simulink model "PatientSIMULATOR_MIMOnoNMB"  (R2022a)
settings: Solver=ode4  StartTime=0.0  StopTime=info.Tsim  FixedStep=0.1  RelTol=1e-15
values from neighbouring files (symbols this model uses):
  condDiscMat = BuildCondendsedMPCmatrices(discreteMat,r,q,F,f,PH)    [MAIN_MIMO.m]    (also in backupMain.m; test.m)
  discreteModel = c2d(continuousModel, info.Ts)    [MAIN_MIMO.m]    (also in backupMain.m; nonLinearPatient_main.m; test.m)
  kalmDiscMat = BuildCondendsedMPCmatrices(discreteMat,r_Kalman,q_Kalman,F,f,PH)    [MAIN_MIMO.m]    (also in test.m)
  PH = 200    [MAIN_MIMO.m]    (also in backupMain.m; nonLinearPatient_main.m; test.m)
  R_KF = 0.001*eye(2)    [MAIN_MIMO.m]    (also in backupMain.m; nonLinearPatient_main.m; test.m)
  wantNoisyBIS = 1    [MAIN_MIMO.m]    (also in backupMain.m; nonLinearPatient_main.m; test.m)
  x_eq = operatingPoint.getstatestruct.signals.values    [MAIN_MIMO.m]    (also in backupMain.m; nonLinearPatient_main.m; test.m)
undefined symbols (not defined in the file or in its folder): continuousModel, Discrete, info, myMPC_dist, op, patient, propofol, RASS, remifentanil, Time
libraries: ctrlSharedLib x3, cstblocks x2
settings Model: Creator=cionescu  LastModifiedBy=user
settings SolverCC: AlgebraicLoopSolver=TrustRegion
settings DataIOCC: SaveState=on  ReturnWorkspaceOutputs=off
settings DebuggingCC: UnconnectedInputMsg=warning  UnconnectedOutputMsg=warning  UnconnectedLineMsg=warning  SFMachineParentedDataDiag=warning  ArithmeticOperatorsInVariantConditions=warning
settings SFSimCC: SimUseLocalCustomCode=off  CustomCodeUndefinedFunction=UseInterfaceOnly
settings RTWCC: RTWUseLocalCustomCode=off  DLArmComputeVersion=19.05
settings CodeAppCC: StateflowObjectComments=on

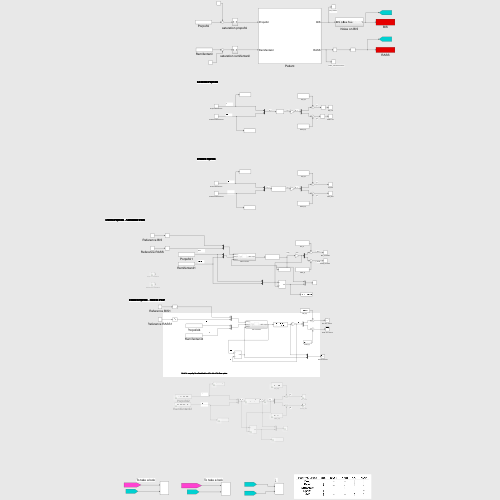
[thumbnail: Simulink's stored preview of the top-level diagram]
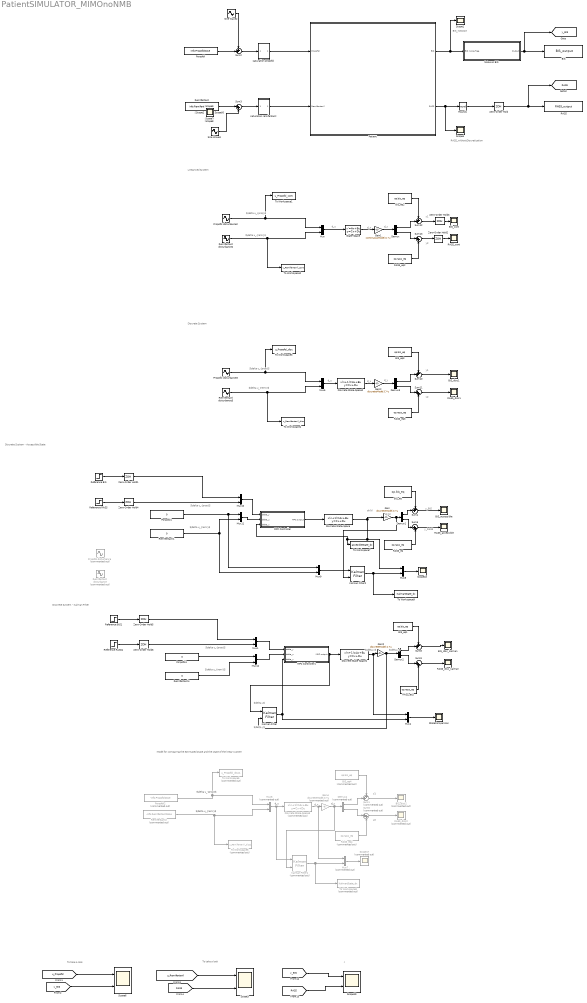
== system PatientSIMULATOR_MIMOnoNMB ==
  note: Model for comparing the estimated state and the state of the linear system
  note: RASS_withoutDiscretization
  note: BIS_noNoise
  note: y2
  note: y1
  note: d_u
  note: d_y
  note: d_x
  note: Linearized System
  note: ↓
  note: To take a look
  note: To take a look
  note: y2
  note: d_y
  note: y1
  note: d_u
  note: d_x
  note: Discrete System
  note: $\delta u_{remi}$
  note: $\delta u_{prop}$
  note: $\delta u_{remi}$
  note: $\delta u_{prop}$
  note: $\delta u_{remi}$
  note: dx(k)
  note: y_RASS
  note: Discrete System - Accessible State
  note: dy(k)
  note: y_BIS
  note: $\delta u_{prop}$
  note: $\delta y$
  note: $\delta x$
  note: $\delta y$
  note: $\delta u$
  note: Discrete System - Kalman Filter
  note: d_u
  note: $\delta u_{remi}$
  note: $\delta u_{prop}$
  note: y1
  note: d_y
  note: y2
  note: d_x
  note: $\delta u_{prop}$
  note: $\delta u_{remi}$
  BIS : ToWorkspace  VariableName=BIS_output  SampleTime=1
      settings: Save2DSignal=2-D array (concatenate along first dimension)
  BIS_accessible : Scope
  BIS_cont : Scope
  BIS_disc1 : Scope
  BIS_disc2 : Scope  Commented=on
  BIS_disc_kalman : Scope
  BIS_eq : Constant  Value=op.bis_eq
  BIS_eq1 : Constant  Value=op.bis_eq
  BIS_eq2 : Constant  Value=op.bis_eq
  BIS_eq3 : Constant  Value=op.bis_eq  SampleTime=info.Ts
  BIS_eq4 : Constant  Commented=on  Value=op.bis_eq  SampleTime=info.Ts
  Demux{,1..3} (4 alike) : Demux  Outputs=2
  Demux4 : Demux  Commented=on  Outputs=2
  Discrete State-Space : DiscreteStateSpace  A=discreteModel.A  B=discreteModel.B  C=eye(size(discreteModel.A))  D=zeros(size(discreteModel.A,1),size(discreteModel.B,2))  InitialCondition=[0,0,0,-0.5584,-2,0,0,0,0,0]'  SampleTime=info.Ts
  Discrete State-Space1 : DiscreteStateSpace  A=discreteModel.A  B=discreteModel.B  C=eye(size(discreteModel.A))  D=zeros(size(discreteModel.A,1),size(discreteModel.B,2))  InitialCondition=[0,0,0,-0.5584,-2,0,0,0,0,0]  SampleTime=info.Ts
  Discrete State-Space2 : DiscreteStateSpace  A=discreteModel.A  B=discreteModel.B  C=eye(size(discreteModel.A))  D=zeros(size(discreteModel.A,1),size(discreteModel.B,2))  InitialCondition=[0,0,0,-0.5584,-2,0,0,0,0,0]'  SampleTime=info.Ts
  Discrete State-Space3 : DiscreteStateSpace  Commented=on  A=discreteModel.A  B=discreteModel.B  C=eye(size(discreteModel.A))  D=zeros(size(discreteModel.A,1),size(discreteModel.B,2))  SampleTime=info.Ts
  Gain : Gain  Gain=discreteModel.C  Multiplication=Matrix(K*u)
  Gain1 : Gain  Gain=continuousModel.C  Multiplication=Matrix(K*u)
  Gain2 : Gain  Gain=discreteModel.C  Multiplication=Matrix(K*u)
  Gain3 : Gain  Gain=discreteModel.C  Multiplication=Matrix(K*u)
  Gain4 : Gain  Commented=on  Gain=discreteModel.C  Multiplication=Matrix(K*u)
  Kalman Filter : ctrlSharedLib/Kalman Filter  TimeDomain=Discrete-Time  UseCurrentEstimator=on  ModelSource=LTI State-Space Variable  ModelSourceVariable=discreteModel  A=0.95  B=1  C=1  D=0  NumberOfStates=1  NumberOfInputs=1  NumberOfOutputs=1  InitialEstimateSource=Dialog  X0=x_eq  P0=10  UseK=off  UseGH=off  NumberOfProcessNoiseInputs=1  G=1  TimeInvariantG=on  H=0  TimeInvariantH=on  Q=Q_KF  TimeInvariantQ=on  R=R_KF  TimeInvariantR=on  N=0  TimeInvariantN=on  AddInputPort=on  AddEnablePort=off  OutputEstimatedY=off  OutputP=off  Ts=-1
  Kalman Filter1 : ctrlSharedLib/Kalman Filter  Commented=on  TimeDomain=Discrete-Time  UseCurrentEstimator=on  ModelSource=LTI State-Space Variable  ModelSourceVariable=discreteModel  A=0.95  B=1  C=1  D=0  NumberOfStates=1  NumberOfInputs=1  NumberOfOutputs=1  InitialEstimateSource=Dialog  X0=[0,0,0,-0.5584,-2,0,0,0,0,0]  P0=10  UseK=off  UseGH=off  NumberOfProcessNoiseInputs=1  G=1  TimeInvariantG=on  H=0  TimeInvariantH=on  Q=Q_KF  TimeInvariantQ=on  R=R_KF  TimeInvariantR=on  N=0  TimeInvariantN=on  AddInputPort=on  AddEnablePort=off  OutputEstimatedY=off  OutputP=off  Ts=-1
  Kalman Filter2 : ctrlSharedLib/Kalman Filter  TimeDomain=Discrete-Time  UseCurrentEstimator=on  ModelSource=LTI State-Space Variable  ModelSourceVariable=discreteModel  A=0.95  B=1  C=1  D=0  NumberOfStates=1  NumberOfInputs=1  NumberOfOutputs=1  InitialEstimateSource=Dialog  X0=[0,0,0,-0.5584,-2,0,0,0,0,0]'  P0=10  UseK=off  UseGH=off  NumberOfProcessNoiseInputs=1  G=1  TimeInvariantG=on  H=0  TimeInvariantH=on  Q=Q_KF  TimeInvariantQ=on  R=R_KF  TimeInvariantR=on  N=0  TimeInvariantN=on  AddInputPort=on  AddEnablePort=off  OutputEstimatedY=off  OutputP=off  Ts=-1
  MPC Controller : Subsystem
  MPC Controller1 : Subsystem
  Mux{,1,4..5,8..12} (9 alike) : Mux  Inputs=2
  Mux6 : Mux  Commented=on  Inputs=2
  Mux7 : Mux  Commented=on  Inputs=2
  Noise on BIS : Subsystem
  Patient : Subsystem
  Porpofol : Constant  Value=info.PropofolDose  SampleTime=info.Ts
  Porpofol1 : Constant  Value=0  SampleTime=info.Ts
  Porpofol2 : Constant  Commented=on  Value=-info.PropofolDose  SampleTime=info.Ts
  Porpofol4 : Constant  Value=0  SampleTime=info.Ts
  Propofol disturbance : Sin  Commented=on  Amplitude=0.3*op.propofol_eq  Frequency=1/500  SampleTime=info.Ts
  Propofol disturbance2 : Sin  Amplitude=0.3*op.propofol_eq  Frequency=1/500  SampleTime=0
  Propofol disturbance3 : Sin  Amplitude=0.3*op.propofol_eq  Frequency=1/500  SampleTime=info.Ts
  RASS : ToWorkspace  VariableName=RASS_output  SampleTime=1
      settings: Save2DSignal=2-D array (concatenate along first dimension)
  RASS_accessible : Scope
  RASS_cont : Scope
  RASS_disc1 : Scope
  RASS_disc2 : Scope  Commented=on
  RASS_disc_kalman : Scope
  RASS_eq : Constant  Value=op.rass_eq
  RASS_eq1 : Constant  Value=op.rass_eq
  RASS_eq2 : Constant  Value=op.rass_eq
  RASS_eq3 : Constant  Value=op.rass_eq  SampleTime=info.Ts
  RASS_eq4 : Constant  Commented=on  Value=op.rass_eq  SampleTime=info.Ts
  Reference BIS : Step  Time=info.T_induction  Before=50  After=0  SampleTime=info.Ts
  Reference BIS1 : Step  Time=info.T_induction  Before=50  After=0  SampleTime=info.Ts
  Reference RASS : Step  Time=info.T_induction  Before=4  After=0  SampleTime=info.Ts
  Reference RASS1 : Step  Time=info.T_induction  Before=4  After=0  SampleTime=info.Ts
  Remifentanil : Constant  Value=info.RemifentanilDose  SampleTime=info.Ts
  Remifentanil disturbance : Sin  Commented=on  Amplitude=0.3*op.remifentanil_eq  Frequency=1/700  SampleTime=info.Ts
  Remifentanil disturbance2 : Sin  Amplitude=0.3*op.remifentanil_eq  Frequency=1/700  SampleTime=0
  Remifentanil disturbance3 : Sin  Amplitude=0.3*op.remifentanil_eq  Frequency=1/700  SampleTime=info.Ts
  Remifentanil1 : Constant  Value=0  SampleTime=info.Ts
  Remifentanil2 : Constant  Commented=on  Value=-info.RemifentanilDose  SampleTime=info.Ts
  Remifentanil4 : Constant  Value=0  SampleTime=info.Ts
  Round1 : Rounding  Operator=round
  Scope{,1..2,4..5,7..16,18} (16 alike) : Scope
  Scope17 : Scope  Commented=on
  Scope19 : Scope  NumInputPorts=2
  Scope3 : Scope  NumInputPorts=2
  Scope6 : Scope  NumInputPorts=2
  Sine Wave2 : Sin  Amplitude=0.3*op.propofol_eq  Frequency=1/500  SampleTime=0
  Sine Wave3 : Sin  Amplitude=0.3*op.remifentanil_eq  Frequency=1/700  SampleTime=0
  State-Space : StateSpace  A=continuousModel.A  B=continuousModel.B  C=eye(size(continuousModel.A))  D=zeros(size(continuousModel.A,1),size(continuousModel.B,2))  InitialCondition=[0,0,0,-0.5584,-2,0,0,0,0,0]'
  StateComparison : Scope
  Sum1 : Sum  Commented=on  Inputs=++|
  Sum{2,4,8,10,12} (5 alike) : Sum  Inputs=++|
  Sum{3,5,9,11,13} (5 alike) : Sum  Inputs=|++
  Sum6 : Sum  Commented=on  Inputs=|++
  To Workspace1 : ToWorkspace  VariableName=u_Propofol_cont  SaveFormat=Structure With Time  SampleTime=-1
      settings: Save2DSignal=2-D array (concatenate along first dimension)
  To Workspace2 : ToWorkspace  VariableName=u_Remifentanil_cont  SaveFormat=Structure With Time  SampleTime=-1
      settings: Save2DSignal=2-D array (concatenate along first dimension)
  To Workspace3 : ToWorkspace  VariableName=u_Propofol_disc  SaveFormat=Structure With Time  SampleTime=info.Ts
      settings: Save2DSignal=2-D array (concatenate along first dimension)
  To Workspace4 : ToWorkspace  VariableName=u_Remifentanil_disc  SaveFormat=Structure With Time  SampleTime=info.Ts
      settings: Save2DSignal=2-D array (concatenate along first dimension)
  To Workspace5 : ToWorkspace  Commented=on  VariableName=u_Propofol_disc1  SaveFormat=Structure With Time  SampleTime=info.Ts
      settings: Save2DSignal=2-D array (concatenate along first dimension)
  To Workspace6 : ToWorkspace  Commented=on  VariableName=u_Remifentanil_disc1  SaveFormat=Structure With Time  SampleTime=info.Ts
      settings: Save2DSignal=2-D array (concatenate along first dimension)
  To Workspace7 : ToWorkspace  VariableName=accesibleState_dx  SaveFormat=Structure With Time  SampleTime=-1
  To Workspace8 : ToWorkspace  Commented=on  VariableName=KalmanState_dx  SaveFormat=Structure With Time  SampleTime=-1
  To Workspace9 : ToWorkspace  VariableName=KalmanState_dx  SaveFormat=Structure With Time  SampleTime=-1
  Zero-Order Hold{,1..6} (7 alike) : ZeroOrderHold  SampleTime=info.Ts
  "saturation propofol " : Subsystem
  saturation remifentanil : Subsystem
  tag scope: RASS=global, y_BIS=global
  wires:
  [u_Propofol] -> Scope6/1
  [y_BIS] -> Scope6/2
  [RASS] -> Scope3/2
  [u_Remifentanil] -> Scope3/1
  Round1/1 -> Zero-Order Hold/1
  [y_BIS] -> Scope19/1
  [RASS] -> Scope19/2
  Zero-Order Hold/1 -> [RASS], RASS/1
  Patient/1(BIS) -> Scope1/1, Noise on BIS/1(BIS noise free)
  Porpofol/1 -> Sum2/2
  "saturation propofol "/1(Out1) -> Patient/1(Propofol)
  Remifentanil/1 -> Sum3/1
  saturation remifentanil/1(Out1) -> Patient/2(Remifentanil)
  Patient/2(RASS) -> Scope4/1, Round1/1
  Noise on BIS/1(Output) -> [y_BIS], BIS/1
  Mux/1 -> State-Space/1
  Propofol disturbance2/1 -> Mux/1, To Workspace1/1
  Remifentanil disturbance2/1 -> To Workspace2/1, Mux/2
  State-Space/1 -> Gain1/1
  Demux/2 -> Sum13/1
  Sine Wave2/1 -> Sum2/1
  Sum2/1 -> "saturation propofol "/1(In1)
  Sine Wave3/1 -> Sum3/2
  Sum3/1 -> saturation remifentanil/1(In1)
  Demux/1 -> Sum12/2
  Gain1/1 -> Demux/1
  BIS_eq2/1 -> Sum12/1
  Sum12/1 -> Zero-Order Hold3/1
  RASS_eq2/1 -> Sum13/2
  Zero-Order Hold3/1 -> BIS_cont/1
  RASS_eq3/1 -> Sum11/2
  BIS_eq3/1 -> Sum10/1
  Propofol disturbance3/1 -> Mux5/1, To Workspace3/1
  Gain3/1 -> Demux3/1
  Demux3/1 -> Sum10/2
  Remifentanil disturbance3/1 -> To Workspace4/1, Mux5/2
  Mux5/1 -> Discrete State-Space2/1
  Demux3/2 -> Sum11/1
  Sum10/1 -> BIS_disc1/1
  Sum11/1 -> RASS_disc1/1
  Sum13/1 -> Zero-Order Hold2/1
  Zero-Order Hold2/1 -> RASS_cont/1
  BIS_eq/1 -> Sum4/1
  Demux1/2 -> Sum5/1
  RASS_eq/1 -> Sum5/2
  Demux1/1 -> Sum4/2
  BIS_eq1/1 -> Sum8/1
  MPC Controller1/1(MPC output) -> Kalman Filter/1, Discrete State-Space1/1
  Sum9/1 -> RASS_disc_kalman/1
  Discrete State-Space1/1 -> Gain2/1, Mux4/1
  RASS_eq1/1 -> Sum9/2
  Gain2/1 -> Demux2/1, Kalman Filter/2
  Sum8/1 -> BIS_disc_kalman/1
  Demux2/2 -> Sum9/1
  Mux4/1 -> StateComparison/1
  Demux2/1 -> Sum8/2
  Gain/1 -> Kalman Filter2/2, Demux1/1
  Discrete State-Space2/1 -> Gain3/1
  Sum5/1 -> RASS_accessible/1
  Sum4/1 -> BIS_accessible/1
  Demux4/2 -> Sum6/1
  Porpofol2/1 -> Mux6/1, To Workspace5/1
  Sum6/1 -> RASS_disc2/1
  Mux6/1 -> Kalman Filter1/1, Discrete State-Space3/1
  Demux4/1 -> Sum1/2
  Discrete State-Space3/1 -> Mux7/1, Gain4/1
  Remifentanil2/1 -> Mux6/2, To Workspace6/1
  Gain4/1 -> Kalman Filter1/2, Demux4/1
  Sum1/1 -> BIS_disc2/1
  RASS_eq4/1 -> Sum6/2
  BIS_eq4/1 -> Sum1/1
  Mux7/1 -> Scope17/1
  Kalman Filter1/1 -> To Workspace8/1, Mux7/2
  Discrete State-Space/1 -> Gain/1, MPC Controller/3(delta_x), To Workspace7/1, Mux8/1
  Mux8/1 -> Scope18/1
  Kalman Filter2/1 -> To Workspace9/1, Mux8/2
  Mux9/1 -> Kalman Filter2/1
  Porpofol1/1 -> Mux9/1, Mux11/1
  Remifentanil1/1 -> Mux9/2, Mux11/2
  Reference BIS/1 -> Zero-Order Hold1/1
  Reference RASS/1 -> Zero-Order Hold4/1
  Zero-Order Hold1/1 -> Mux10/1
  Zero-Order Hold4/1 -> Mux10/2
  Mux10/1 -> MPC Controller/1(delta_y)
  Mux11/1 -> MPC Controller/2(delta_u)
  MPC Controller/1(MPC output) -> Discrete State-Space/1
  Mux12/1 -> MPC Controller1/2(delta_u)
  Mux1/1 -> MPC Controller1/1(delta_y)
  Zero-Order Hold5/1 -> Mux1/1
  Reference BIS1/1 -> Zero-Order Hold5/1
  Remifentanil4/1 -> Mux12/2
  Zero-Order Hold6/1 -> Mux1/2
  Porpofol4/1 -> Mux12/1
  Kalman Filter/1 -> Mux4/2, MPC Controller1/3(delta_x)
  Reference RASS1/1 -> Zero-Order Hold6/1

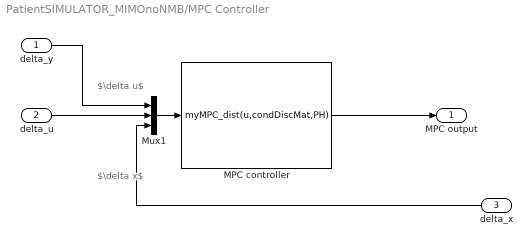
== system PatientSIMULATOR_MIMOnoNMB/MPC Controller ==
  note: $\delta x$
  note: $\delta u$
  delta_y : Inport
  delta_u : Inport  Port=2
  delta_x : Inport  Port=3
  MPC controller : MATLABFcn  MATLABFcn=myMPC_dist(u,condDiscMat,PH)  OutputDimensions=2
  Mux1 : Mux  Inputs=3
  MPC output : Outport
  wires:
  delta_x/1 -> Mux1/3
  Mux1/1 -> MPC controller/1
  MPC controller/1 -> MPC output/1
  delta_u/1 -> Mux1/2
  delta_y/1 -> Mux1/1

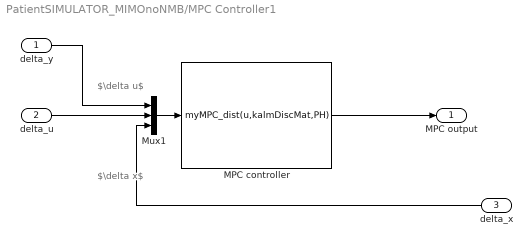
== system PatientSIMULATOR_MIMOnoNMB/MPC Controller1 ==
  note: $\delta x$
  note: $\delta u$
  delta_y : Inport
  delta_u : Inport  Port=2
  delta_x : Inport  Port=3
  MPC controller : MATLABFcn  MATLABFcn=myMPC_dist(u,kalmDiscMat,PH)  OutputDimensions=2
  Mux1 : Mux  Inputs=3
  MPC output : Outport
  wires:
  delta_x/1 -> Mux1/3
  Mux1/1 -> MPC controller/1
  MPC controller/1 -> MPC output/1
  delta_u/1 -> Mux1/2
  delta_y/1 -> Mux1/1

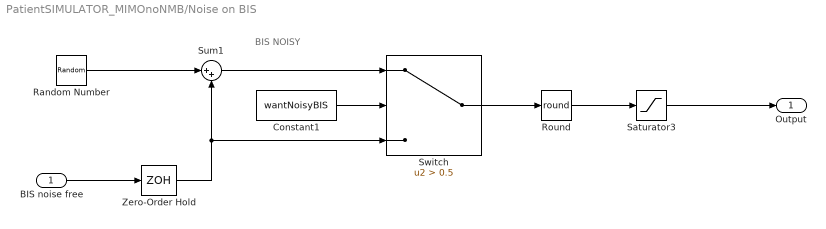
== system PatientSIMULATOR_MIMOnoNMB/Noise on BIS ==
  note: BIS NOISY
  BIS noise free : Inport
  Constant1 : Constant  Value=wantNoisyBIS
  Random Number : RandomNumber  Variance=6.27  SampleTime=info.Ts
  Round : Rounding  Operator=round
  Saturator3 : Saturate  UpperLimit=100  LowerLimit=0
  Sum1 : Sum  Inputs=|++
  Switch : Switch  Criteria=u2 > Threshold  Threshold=0.5  SaturateOnIntegerOverflow=off  InputSameDT=off
  Zero-Order Hold : ZeroOrderHold  SampleTime=info.Ts
  Output : Outport
  wires:
  Round/1 -> Saturator3/1
  Random Number/1 -> Sum1/1
  Constant1/1 -> Switch/2
  Saturator3/1 -> Output/1
  Switch/1 -> Round/1
  BIS noise free/1 -> Zero-Order Hold/1
  Sum1/1 -> Switch/1
  Zero-Order Hold/1 -> Sum1/2, Switch/3

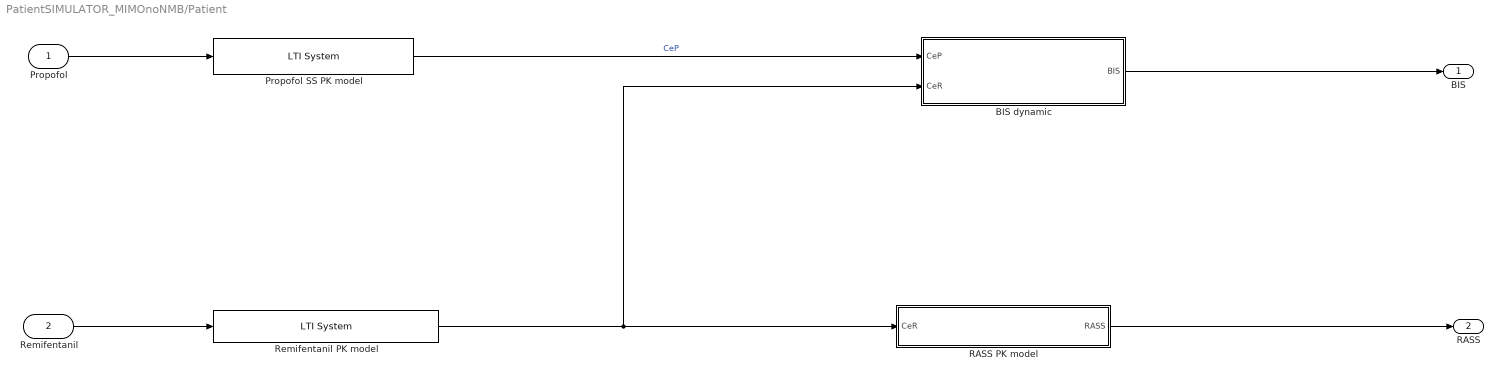
== system PatientSIMULATOR_MIMOnoNMB/Patient ==
  Propofol : Inport
  Remifentanil : Inport  Port=2
  BIS dynamic : Subsystem
  Propofol SS PK model : cstblocks/LTI System  sys=propofol.propSS  IC=0
  RASS PK model : Subsystem
  Remifentanil PK model : cstblocks/LTI System  sys=remifentanil.remiSS  IC=0
  BIS : Outport
  RASS : Outport  Port=2
  wires:
  Propofol SS PK model/1 -> BIS dynamic/1(CeP)  "CeP"
  BIS dynamic/1(BIS) -> BIS/1
  Propofol/1 -> Propofol SS PK model/1
  Remifentanil/1 -> Remifentanil PK model/1
  Remifentanil PK model/1 -> RASS PK model/1(CeR), BIS dynamic/2(CeR)
  RASS PK model/1(RASS) -> RASS/1

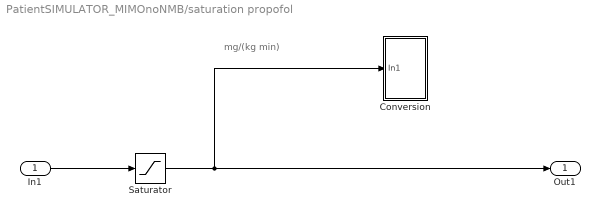
== system PatientSIMULATOR_MIMOnoNMB/saturation propofol  ==
  note: mg/(kg min)
  In1 : Inport
  Conversion : Subsystem
  Saturator : Saturate  UpperLimit=5  LowerLimit=0
  Out1 : Outport
  wires:
  In1/1 -> Saturator/1
  Saturator/1 -> Out1/1, Conversion/1(In1)

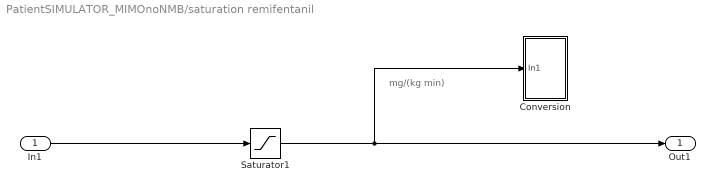
== system PatientSIMULATOR_MIMOnoNMB/saturation remifentanil ==
  note: mg/(kg min)
  In1 : Inport
  "Conversion " : Subsystem
  Saturator1 : Saturate  UpperLimit=2.5  LowerLimit=0
  Out1 : Outport
  wires:
  In1/1 -> Saturator1/1
  Saturator1/1 -> Out1/1, "Conversion "/1(In1)

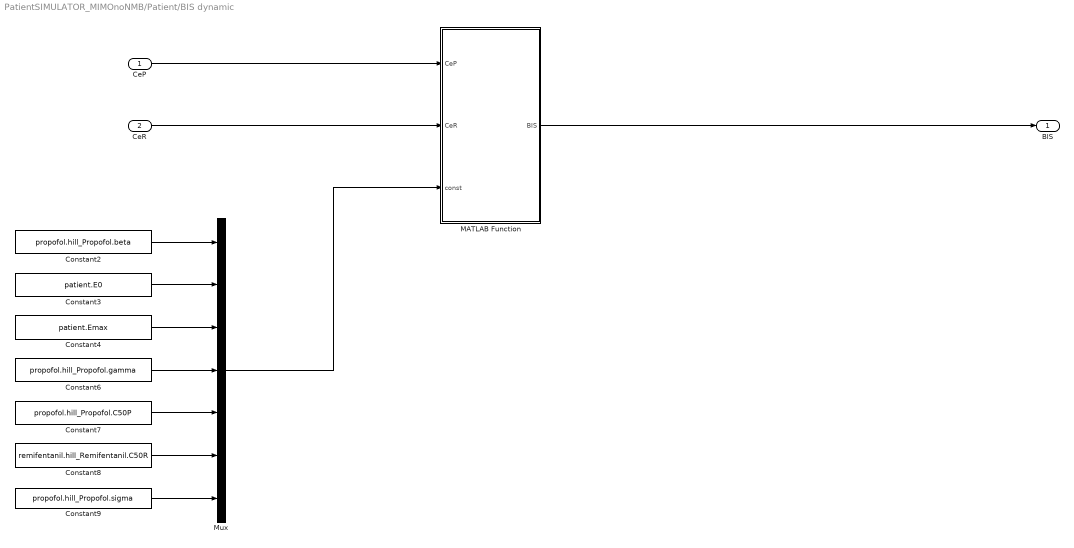
== system PatientSIMULATOR_MIMOnoNMB/Patient/BIS dynamic ==
  CeP : Inport
  CeR : Inport  Port=2
  Constant2 : Constant  Value=propofol.hill_Propofol.beta
  Constant3 : Constant  Value=patient.E0
  Constant4 : Constant  Value=patient.Emax
  Constant6 : Constant  Value=propofol.hill_Propofol.gamma
  Constant7 : Constant  Value=propofol.hill_Propofol.C50P
  Constant8 : Constant  Value=remifentanil.hill_Remifentanil.C50R
  Constant9 : Constant  Value=propofol.hill_Propofol.sigma
  MATLAB Function : MATLAB Function  TreatAsAtomicUnit=on
  Mux : Mux  Inputs=7
  BIS : Outport
  wires:
  Constant9/1 -> Mux/7
  Constant8/1 -> Mux/6
  Constant4/1 -> Mux/3
  Mux/1 -> MATLAB Function/3(const)
  Constant7/1 -> Mux/5
  Constant3/1 -> Mux/2
  Constant6/1 -> Mux/4
  Constant2/1 -> Mux/1
  MATLAB Function/1(BIS) -> BIS/1
  CeP/1 -> MATLAB Function/1(CeP)
  CeR/1 -> MATLAB Function/2(CeR)

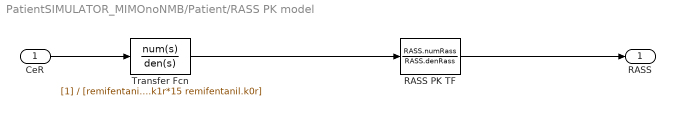
== system PatientSIMULATOR_MIMOnoNMB/Patient/RASS PK model ==
  CeR : Inport
  RASS PK TF : TransferFcn  Numerator=RASS.numRass  Denominator=RASS.denRass
  Transfer Fcn : TransferFcn  Denominator=[remifentanil.k1r*15 remifentanil.k0r]
  RASS : Outport
  wires:
  CeR/1 -> Transfer Fcn/1
  Transfer Fcn/1 -> RASS PK TF/1
  RASS PK TF/1 -> RASS/1

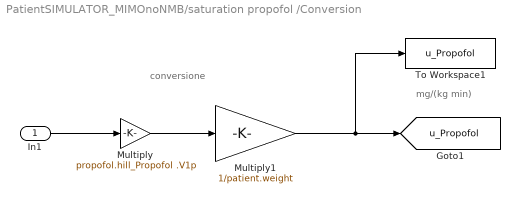
== system PatientSIMULATOR_MIMOnoNMB/saturation propofol /Conversion ==
  note: mg/(kg min)
  note: conversione
  In1 : Inport
  Multiply : Gain  Gain=propofol.hill_Propofol .V1p
  Multiply1 : Gain  Gain=1/patient.weight
  To Workspace1 : ToWorkspace  VariableName=u_Propofol  SaveFormat=Structure With Time  SampleTime=-1
      settings: Save2DSignal=2-D array (concatenate along first dimension)
  tag scope: u_Propofol=global
  wires:
  In1/1 -> Multiply/1
  Multiply/1 -> Multiply1/1
  Multiply1/1 -> To Workspace1/1, [u_Propofol]

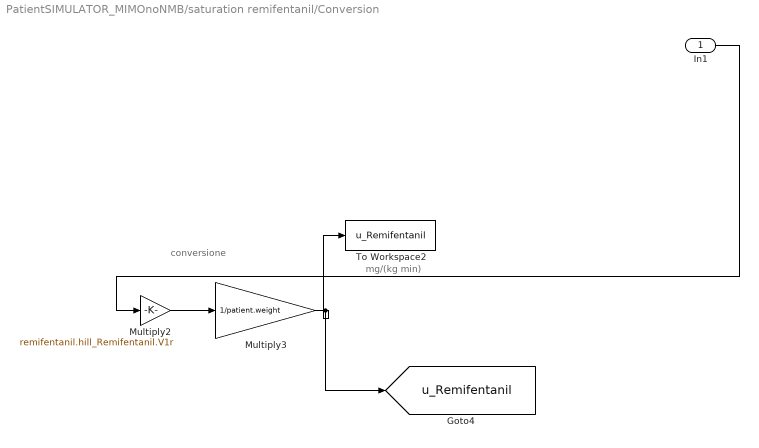
== system PatientSIMULATOR_MIMOnoNMB/saturation remifentanil/Conversion  ==
  note: mg/(kg min)
  note: conversione
  In1 : Inport
  Multiply2 : Gain  Gain=remifentanil.hill_Remifentanil.V1r
  Multiply3 : Gain  Gain=1/patient.weight
  To Workspace2 : ToWorkspace  VariableName=u_Remifentanil  SaveFormat=Structure With Time  SampleTime=-1
      settings: Save2DSignal=2-D array (concatenate along first dimension)
  tag scope: u_Remifentanil=global
  wires:
  Multiply2/1 -> Multiply3/1
  In1/1 -> Multiply2/1
  Multiply3/1 -> To Workspace2/1, [u_Remifentanil]

== matlab function PatientSIMULATOR_MIMOnoNMB/Patient/BIS dynamic/MATLAB Function ==
  data: CeP input; BIS output; CeR input; const input
function BIS = fcn(CeP,CeR, const)

if CeP >=0 && CeR >=0
    %% Constant declaration
    beta = const(1);
    E0 = const(2); %starting effect
%     E0 = const(2)-100; %starting effect
    Emax = const(3); %maximum effect achievable
    gamma = const(4); %sigmoidicity
    C50P = const(5); % half effect concentration
    C50R = const(6); % half effect concentration
    sigma = const(7);% sinergy between prop & rem
    
    %% 2D Calculations
    Uprop=CeP./C50P; Uremi=CeR./C50R;
    BIS=E0 - Emax*((Uprop)+(Uremi)+sigma*(Uprop)*(Uremi))^(gamma)/...
        (1+(Uprop+Uremi+sigma*Uprop*Uremi)^(gamma));

else
    BIS = 100;
end
